simulink model "motor_equations"  (R2013a)
settings: Solver=ode45  StartTime=0.0  StopTime=10.0  RelTol=1e-3
InitFcn:
  | run motor_equations_script
values from neighbouring files (symbols this model uses):
  b = 0.1    [motor_equations_script.m]
  J = 0.01    [motor_equations_script.m]
  Ke = 0.01    [motor_equations_script.m]
  Kt = 0.01    [motor_equations_script.m]
  L = 0.5    [motor_equations_script.m]
  R = 1    [motor_equations_script.m]
settings Model: Creator=ngohara  LastModifiedBy=ngohara

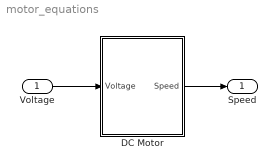
== system motor_equations ==
  "Voltage " : Inport
  DC Motor : Subsystem
  "Speed " : Outport
  wires:
  "Voltage "/1 -> DC Motor/1("Voltage ")
  DC Motor/1("Speed ") -> "Speed "/1

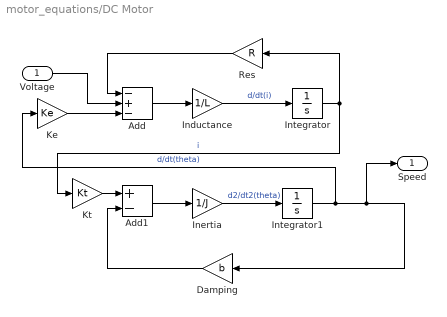
== system motor_equations/DC Motor ==
  "Voltage " : Inport
  Add : Sum  Inputs=-+-
  Add1 : Sum  Inputs=+-
  Damping : Gain  Gain=b
  Inductance : Gain  Gain=1/L
  Inertia : Gain  Gain=1/J
  Integrator : Integrator
  Integrator1 : Integrator
  Ke : Gain  Gain=Ke
  Kt : Gain  Gain=Kt
  Res : Gain  Gain=R
  "Speed " : Outport
  wires:
  Inertia/1 -> Integrator1/1  "d2/dt2(theta)"
  Integrator1/1 -> Ke/1, "Speed "/1, Damping/1  "d/dt(theta)"
  Inductance/1 -> Integrator/1  "d/dt(i)"
  Res/1 -> Add/1
  Kt/1 -> Add1/1
  Ke/1 -> Add/3
  Damping/1 -> Add1/2
  Add/1 -> Inductance/1
  "Voltage "/1 -> Add/2
  Add1/1 -> Inertia/1
  Integrator/1 -> Res/1, Kt/1  "i"
